simulink model "ofur"  (R2018b)
settings: Solver=VariableStepAuto  StartTime=0.0  StopTime=0.01  RelTol=1e-3
libraries: xbsIndex_r4 x105, commanapbnd3 x4
(part 1 of 2)
settings Model: Creator=IRZ  LastModifiedBy=IRZ

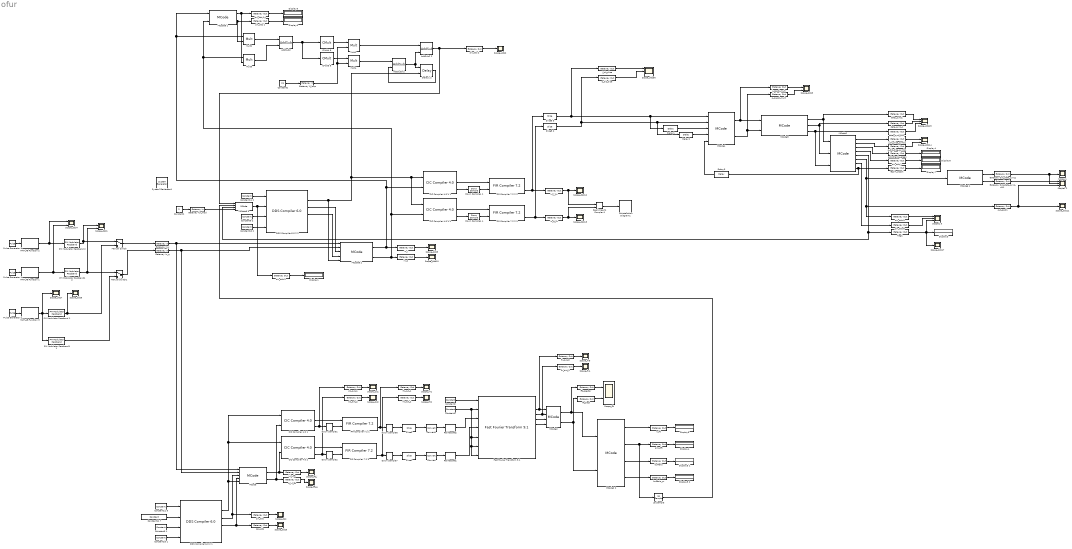
== system ofur ==
  " System Generator1" : xbsIndex_r4/ System Generator  Tag=genX  xilinxfamily=artix7  part=xc7a200t  speed=-3  package=fbg484  synthesis_tool=Vivado  clock_wrapper=Clock Enables  directory=C:/Users/IRZ/AppData/Roaming/Xilinx/Vivado/ofur_24  proj_type=Vivado  Synth_file=Vivado Synthesis Defaults  Impl_file=Vivado Implementation Defaults  testbench=off  simulink_period=1/30.72e6  sysclk_period=32.55  dcm_input_clock_period=10  incr_netlist=off  trim_vbits=Everywhere in SubSystem  dbl_ovrd=According to Block Masks  core_generation=According to Block Masks  run_coregen=off  deprecated_control=off  eval_field=0  block_type=sysgen
  AddSub2 : xbsIndex_r4/AddSub  mode=Subtraction  use_carryin=off  use_carryout=off  en=off  latency=1  precision=Full  arith_type=Unsigned  n_bits=16  bin_pt=14  quantization=Truncate  overflow=Wrap  use_behavioral_HDL=off  hw_selection=Fabric  pipelined=off  dbl_ovrd=off  block_type=addsub
  AddSub2 2 : xbsIndex_r4/AddSub  mode=Addition  use_carryin=off  use_carryout=off  en=off  latency=1  precision=User Defined  arith_type="Signed  (2's comp)"  n_bits=32  bin_pt=32  quantization=Truncate  overflow=Wrap  use_behavioral_HDL=off  hw_selection=Fabric  pipelined=off  dbl_ovrd=off  block_type=addsub
  AddSub3 2 : xbsIndex_r4/AddSub  mode=Addition  use_carryin=off  use_carryout=off  en=off  latency=0  precision=User Defined  arith_type="Signed  (2's comp)"  n_bits=48  bin_pt=48  quantization=Truncate  overflow=Wrap  use_behavioral_HDL=off  hw_selection=Fabric  pipelined=off  dbl_ovrd=off  block_type=addsub
  "CIC Compiler 4.0 1 " : xbsIndex_r4/CIC Compiler 4.0   filter_type=Decimation  number_of_stages=5  differential_delay=1  number_of_channels=1  sample_rate_changes=Fixed  fixed_or_initial_rate=4  minimum_rate=4  maximum_rate=4  ratespecification=Sample_Period  sampleperiod=1  hardwareoversamplingrate=1  quantization=Truncation  output_data_width=24  use_xtreme_dsp_slice=on  use_streaming_interface=on  has_aclken=off  has_aresetn=off  has_dout_tready=off  trim_axipin_name=on  gui_behaviour=Sysgen_GUI  input_data_width=18  ip_name=CIC Compiler  ip_version=4.0  dsptool_ready=true  wrapper_available=true  port_translation_map={ 'aclken' => 'en', 'aresetn' => 'rst' }  ipcore_xco_need_fpga_part=true  ipcore_verbose=false  block_type=cic_compiler_v4_0
  "CIC Compiler 4.0 2 " : xbsIndex_r4/CIC Compiler 4.0   filter_type=Decimation  number_of_stages=5  differential_delay=1  number_of_channels=1  sample_rate_changes=Fixed  fixed_or_initial_rate=4  minimum_rate=4  maximum_rate=4  ratespecification=Sample_Period  sampleperiod=1  hardwareoversamplingrate=1  quantization=Truncation  output_data_width=24  use_xtreme_dsp_slice=on  use_streaming_interface=on  has_aclken=off  has_aresetn=off  has_dout_tready=off  trim_axipin_name=on  gui_behaviour=Sysgen_GUI  input_data_width=18  ip_name=CIC Compiler  ip_version=4.0  dsptool_ready=true  wrapper_available=true  port_translation_map={ 'aclken' => 'en', 'aresetn' => 'rst' }  ipcore_xco_need_fpga_part=true  ipcore_verbose=false  block_type=cic_compiler_v4_0
  CIC Compiler 4.0 4 1 : xbsIndex_r4/CIC Compiler 4.0   filter_type=Decimation  number_of_stages=5  differential_delay=1  number_of_channels=1  sample_rate_changes=Fixed  fixed_or_initial_rate=32  minimum_rate=32  maximum_rate=32  ratespecification=Sample_Period  sampleperiod=1  hardwareoversamplingrate=1  quantization=Truncation  output_data_width=16  use_xtreme_dsp_slice=on  use_streaming_interface=on  has_aclken=off  has_aresetn=off  has_dout_tready=off  trim_axipin_name=on  gui_behaviour=Sysgen_GUI  input_data_width=18  ip_name=CIC Compiler  ip_version=4.0  dsptool_ready=true  wrapper_available=true  port_translation_map={ 'aclken' => 'en', 'aresetn' => 'rst' }  ipcore_xco_need_fpga_part=true  ipcore_verbose=false  block_type=cic_compiler_v4_0
  CIC Compiler 4.0 4 4 : xbsIndex_r4/CIC Compiler 4.0   filter_type=Decimation  number_of_stages=5  differential_delay=1  number_of_channels=1  sample_rate_changes=Fixed  fixed_or_initial_rate=32  minimum_rate=32  maximum_rate=32  ratespecification=Sample_Period  sampleperiod=1  hardwareoversamplingrate=1  quantization=Truncation  output_data_width=16  use_xtreme_dsp_slice=on  use_streaming_interface=on  has_aclken=off  has_aresetn=off  has_dout_tready=off  trim_axipin_name=on  gui_behaviour=Sysgen_GUI  input_data_width=18  ip_name=CIC Compiler  ip_version=4.0  dsptool_ready=true  wrapper_available=true  port_translation_map={ 'aclken' => 'en', 'aresetn' => 'rst' }  ipcore_xco_need_fpga_part=true  ipcore_verbose=false  block_type=cic_compiler_v4_0
  CMult3 5 : xbsIndex_r4/CMult  const=0.00000000010458116751  gui_display_data_type=Fixed-point  const_n_bits=48  const_bin_pt=48  float_type=Single  exp_bits=8  fraction_bits=24  en=off  latency=1  precision=User Defined  arith_type="Signed  (2's comp)"  n_bits=48  bin_pt=48  quantization=Truncate  overflow=Wrap  use_behavioral_HDL=off  mem_type=Distributed RAM  pipeline=off  dbl_ovrd=off  block_type=cmult
  CMult4 5 : xbsIndex_r4/CMult  const=0.0000102265908761675  gui_display_data_type=Fixed-point  const_n_bits=48  const_bin_pt=48  float_type=Single  exp_bits=8  fraction_bits=24  en=off  latency=1  precision=User Defined  arith_type="Signed  (2's comp)"  n_bits=48  bin_pt=48  quantization=Truncate  overflow=Wrap  use_behavioral_HDL=off  mem_type=Distributed RAM  pipeline=off  dbl_ovrd=off  block_type=cmult
  Constant1 : Constant  Value=2
  "Constant1 " : xbsIndex_r4/Constant  const=1.0  gui_display_data_type=Boolean  arith_type=Boolean  n_bits=1  bin_pt=0  preci_type=Single  exp_width=8  frac_width=24  explicit_period=off  period=1/120000  equ=P=C  opselect=C  inp2=PCIN>>17  opr=+  inp1=P  carry=CIN  dbl_ovrd=off  block_type=constant
  Constant10 1 : xbsIndex_r4/Constant  const=1.0  gui_display_data_type=Boolean  arith_type=Boolean  n_bits=16  bin_pt=14  preci_type=Single  exp_width=8  frac_width=24  explicit_period=on  period=1/30.72e6  equ=P=C  opselect=C  inp2=PCIN>>17  opr=+  inp1=P  carry=CIN  dbl_ovrd=off  block_type=constant
  Constant10 2 : xbsIndex_r4/Constant  const=1.0  gui_display_data_type=Boolean  arith_type=Boolean  n_bits=16  bin_pt=14  preci_type=Single  exp_width=8  frac_width=24  explicit_period=on  period=1/30.72e6  equ=P=C  opselect=C  inp2=PCIN>>17  opr=+  inp1=P  carry=CIN  dbl_ovrd=off  block_type=constant
  Constant11 2 : xbsIndex_r4/Constant  const=1.0  gui_display_data_type=Boolean  arith_type=Boolean  n_bits=16  bin_pt=14  preci_type=Single  exp_width=8  frac_width=24  explicit_period=on  period=1/30.72e6  equ=P=C  opselect=C  inp2=PCIN>>17  opr=+  inp1=P  carry=CIN  dbl_ovrd=off  block_type=constant
  Constant11 5 : xbsIndex_r4/Constant  const=1.0  gui_display_data_type=Boolean  arith_type=Boolean  n_bits=16  bin_pt=14  preci_type=Single  exp_width=8  frac_width=24  explicit_period=on  period=1/30.72e6  equ=P=C  opselect=C  inp2=PCIN>>17  opr=+  inp1=P  carry=CIN  dbl_ovrd=off  block_type=constant
  Constant11 7 : xbsIndex_r4/Constant  const=0.03255208333333  gui_display_data_type=Fixed-point  arith_type=Unsigned  n_bits=32  bin_pt=32  preci_type=Single  exp_width=8  frac_width=24  explicit_period=on  period=1/30.72e6  equ=P=C  opselect=C  inp2=PCIN>>17  opr=+  inp1=P  carry=CIN  dbl_ovrd=off  block_type=constant
  Constant2 : Constant  Value=24
  "Constant2 " : xbsIndex_r4/Constant  const=1.0  gui_display_data_type=Fixed-point  arith_type=Unsigned  n_bits=1  bin_pt=0  preci_type=Single  exp_width=8  frac_width=24  explicit_period=off  period=1/120000  equ=P=C  opselect=C  inp2=PCIN>>17  opr=+  inp1=P  carry=CIN  dbl_ovrd=off  block_type=constant
  Constant9 1 : xbsIndex_r4/Constant  const=1.0  gui_display_data_type=Boolean  arith_type=Boolean  n_bits=16  bin_pt=14  preci_type=Single  exp_width=8  frac_width=24  explicit_period=on  period=1/30.72e6  equ=P=C  opselect=C  inp2=PCIN>>17  opr=+  inp1=P  carry=CIN  dbl_ovrd=off  block_type=constant
  Constant9 2 : xbsIndex_r4/Constant  const=1.0  gui_display_data_type=Boolean  arith_type=Boolean  n_bits=16  bin_pt=14  preci_type=Single  exp_width=8  frac_width=24  explicit_period=on  period=1/30.72e6  equ=P=C  opselect=C  inp2=PCIN>>17  opr=+  inp1=P  carry=CIN  dbl_ovrd=off  block_type=constant
  Constellation Diagram1 : ConstellationDiagram
  "Convert " : xbsIndex_r4/Convert  gui_display_data_type=Fixed-point  arith_type="Signed  (2's comp)"  n_bits=21  bin_pt=0  float_type=Single  exp_bits=8  fraction_bits=24  quantization=Truncate  overflow=Wrap  en=off  latency=0  pipeline=off  dbl_ovrd=off  block_type=convert
  "Convert1 " : xbsIndex_r4/Convert  gui_display_data_type=Fixed-point  arith_type="Signed  (2's comp)"  n_bits=21  bin_pt=0  float_type=Single  exp_bits=8  fraction_bits=24  quantization=Truncate  overflow=Wrap  en=off  latency=0  pipeline=off  dbl_ovrd=off  block_type=convert
  DDS Compiler 6.0 2 1 : xbsIndex_r4/DDS Compiler 6.0   partspresent=Phase_Generator_and_SIN_COS_LUT  dds_clock_rate=30.72  channels=1  mode_of_operation=Standard  modulus=9  parameter_entry=Hardware_Parameters  spurious_free_dynamic_range=45  frequency_resolution=0.4  noise_shaping=None  phase_width=32  output_width=12  output_selection=Sine_and_Cosine  negative_sine=on  negative_cosine=on  amplitude_mode=Full_Range  memory_type=Auto  optimization_goal=Auto  dsp48_use=Minimal  resync=off  latency_configuration=Auto  latency=1  has_phase_out=on  has_aclken=off  has_aresetn=off  explicit_period=on  period=1/30.72e6  data_has_tlast=Not_Required  has_tready=on  s_phase_has_tuser=Not_Required  m_data_has_tuser=Not_Required  m_phase_has_tuser=Not_Required  s_phase_tuser_width=1  output_form=Twos_Complement  s_config_sync_mode=On_Vector  phase_increment=Streaming  output_frequency1=0  output_frequency2=0  output_frequency3=0  output_frequency4=0  output_frequency5=0  output_frequency6=0  output_frequency7=0  output_frequency8=0  output_frequency9=0  output_frequency10=0  output_frequency11=0  output_frequency12=0  output_frequency13=0  output_frequency14=0  output_frequency15=0  output_frequency16=0  pinc1='0'  pinc2='0'  pinc3='0'  pinc4='0'  pinc5='0'  pinc6='0'  pinc7='0'  pinc8='0'  pinc9='0'  pinc10='0'  pinc11='0'  pinc12='0'  pinc13='0'  pinc14='0'  pinc15='0'  pinc16='0'  phase_offset=Fixed  phase_offset_angles1=0  phase_offset_angles2=0  phase_offset_angles3=0  phase_offset_angles4=0  phase_offset_angles5=0  phase_offset_angles6=0  phase_offset_angles7=0  phase_offset_angles8=0  phase_offset_angles9=0  phase_offset_angles10=0  phase_offset_angles11=0  phase_offset_angles12=0  phase_offset_angles13=0  phase_offset_angles14=0  phase_offset_angles15=0  phase_offset_angles16=0  poff1='0'  poff2='0'  poff3='0'  poff4='0'  poff5='0'  poff6='0'  poff7='0'  poff8='0'  poff9='0'  poff10='0'  poff11='0'  poff12='0'  poff13='0'  poff14='0'  poff15='0'  poff16='0'  trim_axipin_name=on  simulation_type=hybrid_sim  simulation_model=sysgen:xddsv6_0_cmodel  data_path_portlist={ 's_axis_config_tdata_poff', 's_axis_config_tdata_chan0_poff', 's_axis_config_tdata_pinc', 's_axis_config_tdata_chan0_pinc', 's_axis_phase_tdata_resync', 's_axis_phase_tdata_chan0_resync', 's_axis_phase_tdata_poff', 's_axis_phase_tdata_chan0_poff', 's_axis_phase_tdata_pinc', 's_axis_phase_tdata_chan0_pinc', 's_axis_phase_tdata_phase_in', 'm_axis_data_tdata_sine', 'm_axis_data_tdata_chan0_sine', 'm_axis_data_tdata_cosine', 'm_axis_data_tdata_chan0_cosine', 'm_axis_phase_tdata_phase_out', 'm_axis_phase_tdata_chan0_phase_out'}  por_mode=false  gui_behaviour=Sysgen  ip_name=DDS Compiler  ip_version=6.0  dsptool_ready=true  wrapper_available=true  port_translation_map={ 'aclken' => 'en', 'aresetn' => 'rst' }  ipcore_usecache=true  ipcore_useipmodelcache=true  ipcore_xco_need_fpga_part=true  ipcore_verbose=false  block_type=dds_compiler_v6_0
  DDS Compiler 6.0 2 2 : xbsIndex_r4/DDS Compiler 6.0   partspresent=Phase_Generator_and_SIN_COS_LUT  dds_clock_rate=30.72  channels=1  mode_of_operation=Standard  modulus=9  parameter_entry=Hardware_Parameters  spurious_free_dynamic_range=45  frequency_resolution=0.4  noise_shaping=None  phase_width=32  output_width=12  output_selection=Sine_and_Cosine  negative_sine=on  negative_cosine=on  amplitude_mode=Full_Range  memory_type=Auto  optimization_goal=Auto  dsp48_use=Minimal  resync=off  latency_configuration=Auto  latency=1  has_phase_out=on  has_aclken=off  has_aresetn=off  explicit_period=on  period=1/30.72e6  data_has_tlast=Not_Required  has_tready=on  s_phase_has_tuser=Not_Required  m_data_has_tuser=Not_Required  m_phase_has_tuser=Not_Required  s_phase_tuser_width=1  output_form=Twos_Complement  s_config_sync_mode=On_Vector  phase_increment=Streaming  output_frequency1=0  output_frequency2=0  output_frequency3=0  output_frequency4=0  output_frequency5=0  output_frequency6=0  output_frequency7=0  output_frequency8=0  output_frequency9=0  output_frequency10=0  output_frequency11=0  output_frequency12=0  output_frequency13=0  output_frequency14=0  output_frequency15=0  output_frequency16=0  pinc1='0'  pinc2='0'  pinc3='0'  pinc4='0'  pinc5='0'  pinc6='0'  pinc7='0'  pinc8='0'  pinc9='0'  pinc10='0'  pinc11='0'  pinc12='0'  pinc13='0'  pinc14='0'  pinc15='0'  pinc16='0'  phase_offset=Fixed  phase_offset_angles1=0  phase_offset_angles2=0  phase_offset_angles3=0  phase_offset_angles4=0  phase_offset_angles5=0  phase_offset_angles6=0  phase_offset_angles7=0  phase_offset_angles8=0  phase_offset_angles9=0  phase_offset_angles10=0  phase_offset_angles11=0  phase_offset_angles12=0  phase_offset_angles13=0  phase_offset_angles14=0  phase_offset_angles15=0  phase_offset_angles16=0  poff1='0'  poff2='0'  poff3='0'  poff4='0'  poff5='0'  poff6='0'  poff7='0'  poff8='0'  poff9='0'  poff10='0'  poff11='0'  poff12='0'  poff13='0'  poff14='0'  poff15='0'  poff16='0'  trim_axipin_name=on  simulation_type=hybrid_sim  simulation_model=sysgen:xddsv6_0_cmodel  data_path_portlist={ 's_axis_config_tdata_poff', 's_axis_config_tdata_chan0_poff', 's_axis_config_tdata_pinc', 's_axis_config_tdata_chan0_pinc', 's_axis_phase_tdata_resync', 's_axis_phase_tdata_chan0_resync', 's_axis_phase_tdata_poff', 's_axis_phase_tdata_chan0_poff', 's_axis_phase_tdata_pinc', 's_axis_phase_tdata_chan0_pinc', 's_axis_phase_tdata_phase_in', 'm_axis_data_tdata_sine', 'm_axis_data_tdata_chan0_sine', 'm_axis_data_tdata_cosine', 'm_axis_data_tdata_chan0_cosine', 'm_axis_phase_tdata_phase_out', 'm_axis_phase_tdata_chan0_phase_out'}  por_mode=false  gui_behaviour=Sysgen  ip_name=DDS Compiler  ip_version=6.0  dsptool_ready=true  wrapper_available=true  port_translation_map={ 'aclken' => 'en', 'aresetn' => 'rst' }  ipcore_usecache=true  ipcore_useipmodelcache=true  ipcore_xco_need_fpga_part=true  ipcore_verbose=false  block_type=dds_compiler_v6_0
  Delay1 : xbsIndex_r4/Delay  rst=off  infoeditControl=Selection of Reset will increase slice count due to use of real FFs and instead of SRLs  en=off  latency=60  reg_retiming=off  dbl_ovrd=off  block_type=delay
  Delay1 2 : xbsIndex_r4/Delay  rst=off  infoeditControl=Selection of Reset will increase slice count due to use of real FFs and instead of SRLs  en=on  latency=1  reg_retiming=off  dbl_ovrd=off  block_type=delay
  Delay2 : xbsIndex_r4/Delay  rst=off  infoeditControl=Selection of Reset will increase slice count due to use of real FFs and instead of SRLs  en=off  latency=60  reg_retiming=off  dbl_ovrd=off  block_type=delay
  Delay3 : xbsIndex_r4/Delay  rst=off  infoeditControl=Selection of Reset will increase slice count due to use of real FFs and instead of SRLs  en=off  latency=1  reg_retiming=off  dbl_ovrd=off  block_type=delay
  Display{1,3..8} (7 alike) : Display
  "Display4 " : Display
  "Display5 " : Display
  Display5 1 : Display
  Display5 2 : Display
  "Down Sample1 " : xbsIndex_r4/Down Sample  sample_ratio=4  sample_phase="Last Value of Frame  (most efficient)"  en=off  rst=off  latency=1  dbl_ovrd=off  block_type=dsamp
  "Down Sample2 " : xbsIndex_r4/Down Sample  sample_ratio=4  sample_phase="Last Value of Frame  (most efficient)"  en=off  rst=off  latency=1  dbl_ovrd=off  block_type=dsamp
  Down Sample4 1 : xbsIndex_r4/Down Sample  sample_ratio=32  sample_phase="Last Value of Frame  (most efficient)"  en=off  rst=off  latency=1  dbl_ovrd=off  block_type=dsamp
  Down Sample4 4 : xbsIndex_r4/Down Sample  sample_ratio=32  sample_phase="Last Value of Frame  (most efficient)"  en=off  rst=off  latency=1  dbl_ovrd=off  block_type=dsamp
  "Down Sample6 " : xbsIndex_r4/Down Sample  sample_ratio=4  sample_phase="Last Value of Frame  (most efficient)"  en=off  rst=off  latency=1  dbl_ovrd=off  block_type=dsamp
  "Down Sample7 " : xbsIndex_r4/Down Sample  sample_ratio=4  sample_phase="Last Value of Frame  (most efficient)"  en=off  rst=off  latency=1  dbl_ovrd=off  block_type=dsamp
  "FIR Compiler 7.2 1 " : xbsIndex_r4/FIR Compiler 7.2   coefficientvector=[5961,-4341,-5200,5397,4251,-6331,-3141,7100,1875,-7671,-458,8028,-1084,-8145,2709,7981,-4390,-7515,6071,6714,-7711,-5578,9238,4098,-10576,-2278,11650,136,-12393,2277,12717,-4911,-12561,7674,11849,-10487,-10548,13229,8632,-15771,-6099,17971,2967,-19698,699,20806,-4819,-21177,9255,20681,-13870,-19237,18484,16792,-22893,-13332,26871,8872,-30202,-3496,32654,-2687,-34033,9480,34134,-16674,-32809,24007,29954,-31182,-25527,37863,19534,-43720,-12068,48399,3266,-51603,6615,53018,-17279,-52399,28360,49556,-39446,-44391,50062,36877,-59727,-27101,67922,15214,-74196,-1526,78087,-13579,-79202,29613,77220,-46023,-71936,62164,63244,-77368,-51198,90890,35929,-102064,-17776,110212,-2802,-114730,25190,115084,-48675,-110890,72410,101880,-95502,-88017,116918,69351,-135693,-46197,150834,19045,-161429,11387,166618,-44226,-165712,78400,158145,-112759,-143659,145915,122105,-176513,-93664,203106,58734,-224327,-18056,238810,-27410,-245362,76380,242864,-127466,-230591,178883,207912,-228803,-174609,275166,130682,-315950,-76603,348997,13114,-372286,58521,383660,-136955,-381405,220191,363720,-306141,-329247,392180,276603,-475673,-204895,553510,113191,-622681,-1152,679399,-132151,-720279,287147,740942,-465392,-737162,668670,702872,-901701,-631137,1172158,510308,-1497574,-323934,1911126,37391,-2496341,416174,3480027,-1210770,-5782518,2698242,16777215,16777215,2698242,-5782518,-1210770,3480027,416174,-2496341,37391,1911126,-323934,-1497574,510308,1172158,-631137,-901701,702872,668670,-737162,-465392,740942,287147,-720279,-132151,679399,-1152,-622681,113191,553510,-204895,-475673,276603,392180,-329247,-306141,363720,220191,-381405,-136955,383660,58521,-372286,13114,348997,-76603,-315950,130682,275166,-174609,-228803,207912,178883,-230591,-127466,242864,76380,-245362,-27410,238810,-18056,-224327,58734,203106,-93664,-176513,122105,145915,-143659,-112759,158145,78400,-165712,-44226,166618,11387,-161429,19045,150834,-46197,-135693,69351,116918,-88017,-95502,101880,72410,-110890,-48675,115084,25190,-114730,-2802,110212,-17776,-102064,35929,90890,-51198,-77368,63244,62164,-71936,-46023,77220,29613,-79202,-13579,78087,-1526,-74196,15214,67922,-27101,-59727,36877,50062,-44391,-39446,49556,28360,-52399,-17279,53018,6615,-51603,3266,48399,-12068,-43720,19534,37863,-25527,-31182,29954,24007,-32809,-16674,34134,9480,-34033,-2687,32654,-3496,-30202,8872,26871,-13332,-22893,16792,18484,-19237,-13870,20681,9255,-21177,-4819,20806,699,-19698,2967,17971,-6099,-15771,8632,13229,-10548,-10487,11849,7674,-12561,-4911,12717,2277,-12393,136,11650,-2278,-10576,4098,9238,-5578,-7711,6714,6071,-7515,-4390,7981,2709,-8145,-1084,8028,-458,-7671,1875,7100,-3141,-6331,4251,5397,-5200,-4341,5961]  coefficient_sets=1  coefficient_reload=off  filter_type=Single_Rate  rate_change_type=Integer  interpolation_rate=1  decimation_rate=1  zero_pack_factor=1  channel_sequence=Basic  number_channels=1  pattern_list='P4-0,P4-1,P4-2,P4-3,P4-4'  number_paths=1  ratespecification=Input_Sample_Period  sampleperiod=4  hardwareoversamplingrate=1  coefficient_sign=Signed  quantization=Integer_Coefficients  coefficient_width=25  bestprecision=off  coefficient_fractional_bits=0  coefficient_structure=Inferred  output_rounding_mode=Truncate_LSBs  output_width=24  filter_architecture=Systolic_Multiply_Accumulate  optimization_goal=Area  optimization_list='None'  data_buffer_type=Automatic  coefficient_buffer_type=Automatic  input_buffer_type=Automatic  output_buffer_type=Automatic  preference_for_other_storage=Automatic  multi_column_support=Automatic  columnconfig='51'  inter_column_pipe_length=4  data_has_tlast=Not_Required  m_data_has_tready=off  s_data_has_fifo=off  s_data_has_tuser=Not_Required  m_data_has_tuser=Not_Required  s_config_sync_mode=On_Vector  s_config_method=Single  num_reload_slots=1  has_aclken=off  has_aresetn=off  infoeditControl=ARESETn must be asserted for a minimum of 2 cycles  reset_data_vector=on  trim_axipin_name=on  simulation_type=hybrid_sim  simulation_model=sysgen:xfirv7_2_cmodel  data_path_portlist={ 's_axis_data_tdata', 'm_axis_data_tdata' }  passband_min=0.0  passband_max=0.5  stopband_min=0.5  stopband_max=1.0  filter_selection=1  gui_behaviour='Sysgen_GUI'  data_sign=Signed  data_width=16  data_fractional_bits=0  data_tuser_width=1  wrapper_available=true  ip_wrap_arbitrary_binary_point=true  ip_name=FIR Compiler  ip_version=7.2  dsptool_ready=true  ipcore_usecache=true  ipcore_useipmodelcache=true  port_translation_map={ 'aclken' => 'en', 'aresetn' => 'rst' }  run_core_at_system_period=true  ipcore_xco_need_fpga_part=true  block_type=fir_compiler_v7_2
      settings: infoedit=Maximum Possible : Maximizes oversampling rate. Abstracted input handshake (no s_data_tvalid) and automatic rate propagation.<br>Hardware Oversampling Rate : Specifies oversampling rate relative to the input sample period. Abstracted input handshake (no s_data_tvalid) and automatic rate propagation.<br>Input/Output Sample Period : Specifies absolute oversampling rate. No input handshake abstraction (exposes s_data_tvalid) and no rate propagation.
  FIR Compiler 7.2 2 1 : xbsIndex_r4/FIR Compiler 7.2   coefficientvector=[5553,-5324,-4273,6479,2702,-7305,-920,7729,-1006,-7701,3003,7201,-4966,-6223,6772,4761,-8314,-2856,9463,560,-10121,2017,10174,-4751,-9540,7488,8172,-10055,-6076,12244,3285,-13863,90,14710,-3911,-14639,7955,13523,-11964,-11299,15648,7970,-18710,-3641,20835,-1519,-21758,7231,21238,-13176,-19143,18942,15423,-24088,-10141,28160,3476,-30743,4251,31459,-12621,-30047,21090,26330,-29083,-20322,35967,12188,-41120,-2270,43970,-8936,-44066,20767,41089,-32467,-34935,43163,25668,-52014,-13621,58198,-650,-61006,16364,59879,-32580,-54501,48204,44804,-62111,-31063,73124,13805,-80206,6116,82482,-27581,-79334,49244,70445,-69637,-55886,87221,36094,-100558,-11978,108295,-15238,-109384,43981,103126,-72441,-89280,98635,68072,-120580,-40278,136365,7130,-144406,29567,143406,-67681,-132608,104757,111814,-138224,-81521,165478,42865,-184127,2310,192056,-51669,-187798,102250,170439,-150824,-139900,193936,96894,-228227,-43078,250533,-19090,-258224,86280,249201,-154701,-222419,219925,177699,-277402,-116076,322477,39610,-350898,48399,358869,-143713,-343561,240967,302909,-334404,-236394,417533,144637,-483910,-29968,526925,-104076,-540617,252289,519407,-408479,-459016,564715,355472,-712754,-206430,842864,9618,-945294,236166,1008549,-533823,-1020728,888019,965947,-1312331,-824719,1835158,561006,-2534935,-109960,3632892,-689814,-6037165,2102535,16777215,16777215,2102535,-6037165,-689814,3632892,-109960,-2534935,561006,1835158,-824719,-1312331,965947,888019,-1020728,-533823,1008549,236166,-945294,9618,842864,-206430,-712754,355472,564715,-459016,-408479,519407,252289,-540617,-104076,526925,-29968,-483910,144637,417533,-236394,-334404,302909,240967,-343561,-143713,358869,48399,-350898,39610,322477,-116076,-277402,177699,219925,-222419,-154701,249201,86280,-258224,-19090,250533,-43078,-228227,96894,193936,-139900,-150824,170439,102250,-187798,-51669,192056,2310,-184127,42865,165478,-81521,-138224,111814,104757,-132608,-67681,143406,29567,-144406,7130,136365,-40278,-120580,68072,98635,-89280,-72441,103126,43981,-109384,-15238,108295,-11978,-100558,36094,87221,-55886,-69637,70445,49244,-79334,-27581,82482,6116,-80206,13805,73124,-31063,-62111,44804,48204,-54501,-32580,59879,16364,-61006,-650,58198,-13621,-52014,25668,43163,-34935,-32467,41089,20767,-44066,-8936,43970,-2270,-41120,12188,35967,-20322,-29083,26330,21090,-30047,-12621,31459,4251,-30743,3476,28160,-10141,-24088,15423,18942,-19143,-13176,21238,7231,-21758,-1519,20835,-3641,-18710,7970,15648,-11299,-11964,13523,7955,-14639,-3911,14710,90,-13863,3285,12244,-6076,-10055,8172,7488,-9540,-4751,10174,2017,-10121,560,9463,-2856,-8314,4761,6772,-6223,-4966,7201,3003,-7701,-1006,7729,-920,-7305,2702,6479,-4273,-5324,5553]  coefficient_sets=1  coefficient_reload=off  filter_type=Single_Rate  rate_change_type=Integer  interpolation_rate=1  decimation_rate=1  zero_pack_factor=1  channel_sequence=Basic  number_channels=1  pattern_list='P4-0,P4-1,P4-2,P4-3,P4-4'  number_paths=1  ratespecification=Input_Sample_Period  sampleperiod=32  hardwareoversamplingrate=1  coefficient_sign=Signed  quantization=Integer_Coefficients  coefficient_width=25  bestprecision=off  coefficient_fractional_bits=0  coefficient_structure=Inferred  output_rounding_mode=Truncate_LSBs  output_width=16  filter_architecture=Systolic_Multiply_Accumulate  optimization_goal=Area  optimization_list='None'  data_buffer_type=Automatic  coefficient_buffer_type=Automatic  input_buffer_type=Automatic  output_buffer_type=Automatic  preference_for_other_storage=Automatic  multi_column_support=Automatic  columnconfig='7'  inter_column_pipe_length=4  data_has_tlast=Not_Required  m_data_has_tready=off  s_data_has_fifo=off  s_data_has_tuser=Not_Required  m_data_has_tuser=Not_Required  s_config_sync_mode=On_Vector  s_config_method=Single  num_reload_slots=1  has_aclken=off  has_aresetn=off  infoeditControl=ARESETn must be asserted for a minimum of 2 cycles  reset_data_vector=on  trim_axipin_name=on  simulation_type=hybrid_sim  simulation_model=sysgen:xfirv7_2_cmodel  data_path_portlist={ 's_axis_data_tdata', 'm_axis_data_tdata' }  passband_min=0.0  passband_max=0.5  stopband_min=0.5  stopband_max=1.0  filter_selection=1  gui_behaviour='Sysgen_GUI'  data_sign=Signed  data_width=16  data_fractional_bits=0  data_tuser_width=1  wrapper_available=true  ip_wrap_arbitrary_binary_point=true  ip_name=FIR Compiler  ip_version=7.2  dsptool_ready=true  ipcore_usecache=true  ipcore_useipmodelcache=true  port_translation_map={ 'aclken' => 'en', 'aresetn' => 'rst' }  run_core_at_system_period=true  ipcore_xco_need_fpga_part=true  block_type=fir_compiler_v7_2
      settings: infoedit=Maximum Possible : Maximizes oversampling rate. Abstracted input handshake (no s_data_tvalid) and automatic rate propagation.<br>Hardware Oversampling Rate : Specifies oversampling rate relative to the input sample period. Abstracted input handshake (no s_data_tvalid) and automatic rate propagation.<br>Input/Output Sample Period : Specifies absolute oversampling rate. No input handshake abstraction (exposes s_data_tvalid) and no rate propagation.
  FIR Compiler 7.2 2 4 : xbsIndex_r4/FIR Compiler 7.2   coefficientvector=[5553,-5324,-4273,6479,2702,-7305,-920,7729,-1006,-7701,3003,7201,-4966,-6223,6772,4761,-8314,-2856,9463,560,-10121,2017,10174,-4751,-9540,7488,8172,-10055,-6076,12244,3285,-13863,90,14710,-3911,-14639,7955,13523,-11964,-11299,15648,7970,-18710,-3641,20835,-1519,-21758,7231,21238,-13176,-19143,18942,15423,-24088,-10141,28160,3476,-30743,4251,31459,-12621,-30047,21090,26330,-29083,-20322,35967,12188,-41120,-2270,43970,-8936,-44066,20767,41089,-32467,-34935,43163,25668,-52014,-13621,58198,-650,-61006,16364,59879,-32580,-54501,48204,44804,-62111,-31063,73124,13805,-80206,6116,82482,-27581,-79334,49244,70445,-69637,-55886,87221,36094,-100558,-11978,108295,-15238,-109384,43981,103126,-72441,-89280,98635,68072,-120580,-40278,136365,7130,-144406,29567,143406,-67681,-132608,104757,111814,-138224,-81521,165478,42865,-184127,2310,192056,-51669,-187798,102250,170439,-150824,-139900,193936,96894,-228227,-43078,250533,-19090,-258224,86280,249201,-154701,-222419,219925,177699,-277402,-116076,322477,39610,-350898,48399,358869,-143713,-343561,240967,302909,-334404,-236394,417533,144637,-483910,-29968,526925,-104076,-540617,252289,519407,-408479,-459016,564715,355472,-712754,-206430,842864,9618,-945294,236166,1008549,-533823,-1020728,888019,965947,-1312331,-824719,1835158,561006,-2534935,-109960,3632892,-689814,-6037165,2102535,16777215,16777215,2102535,-6037165,-689814,3632892,-109960,-2534935,561006,1835158,-824719,-1312331,965947,888019,-1020728,-533823,1008549,236166,-945294,9618,842864,-206430,-712754,355472,564715,-459016,-408479,519407,252289,-540617,-104076,526925,-29968,-483910,144637,417533,-236394,-334404,302909,240967,-343561,-143713,358869,48399,-350898,39610,322477,-116076,-277402,177699,219925,-222419,-154701,249201,86280,-258224,-19090,250533,-43078,-228227,96894,193936,-139900,-150824,170439,102250,-187798,-51669,192056,2310,-184127,42865,165478,-81521,-138224,111814,104757,-132608,-67681,143406,29567,-144406,7130,136365,-40278,-120580,68072,98635,-89280,-72441,103126,43981,-109384,-15238,108295,-11978,-100558,36094,87221,-55886,-69637,70445,49244,-79334,-27581,82482,6116,-80206,13805,73124,-31063,-62111,44804,48204,-54501,-32580,59879,16364,-61006,-650,58198,-13621,-52014,25668,43163,-34935,-32467,41089,20767,-44066,-8936,43970,-2270,-41120,12188,35967,-20322,-29083,26330,21090,-30047,-12621,31459,4251,-30743,3476,28160,-10141,-24088,15423,18942,-19143,-13176,21238,7231,-21758,-1519,20835,-3641,-18710,7970,15648,-11299,-11964,13523,7955,-14639,-3911,14710,90,-13863,3285,12244,-6076,-10055,8172,7488,-9540,-4751,10174,2017,-10121,560,9463,-2856,-8314,4761,6772,-6223,-4966,7201,3003,-7701,-1006,7729,-920,-7305,2702,6479,-4273,-5324,5553]  coefficient_sets=1  coefficient_reload=off  filter_type=Single_Rate  rate_change_type=Integer  interpolation_rate=1  decimation_rate=1  zero_pack_factor=1  channel_sequence=Basic  number_channels=1  pattern_list='P4-0,P4-1,P4-2,P4-3,P4-4'  number_paths=1  ratespecification=Input_Sample_Period  sampleperiod=32  hardwareoversamplingrate=1  coefficient_sign=Signed  quantization=Integer_Coefficients  coefficient_width=25  bestprecision=off  coefficient_fractional_bits=0  coefficient_structure=Inferred  output_rounding_mode=Truncate_LSBs  output_width=16  filter_architecture=Systolic_Multiply_Accumulate  optimization_goal=Area  optimization_list='None'  data_buffer_type=Automatic  coefficient_buffer_type=Automatic  input_buffer_type=Automatic  output_buffer_type=Automatic  preference_for_other_storage=Automatic  multi_column_support=Automatic  columnconfig='7'  inter_column_pipe_length=4  data_has_tlast=Not_Required  m_data_has_tready=off  s_data_has_fifo=off  s_data_has_tuser=Not_Required  m_data_has_tuser=Not_Required  s_config_sync_mode=On_Vector  s_config_method=Single  num_reload_slots=1  has_aclken=off  has_aresetn=off  infoeditControl=ARESETn must be asserted for a minimum of 2 cycles  reset_data_vector=on  trim_axipin_name=on  simulation_type=hybrid_sim  simulation_model=sysgen:xfirv7_2_cmodel  data_path_portlist={ 's_axis_data_tdata', 'm_axis_data_tdata' }  passband_min=0.0  passband_max=0.5  stopband_min=0.5  stopband_max=1.0  filter_selection=1  gui_behaviour='Sysgen_GUI'  data_sign=Signed  data_width=16  data_fractional_bits=0  data_tuser_width=1  wrapper_available=true  ip_wrap_arbitrary_binary_point=true  ip_name=FIR Compiler  ip_version=7.2  dsptool_ready=true  ipcore_usecache=true  ipcore_useipmodelcache=true  port_translation_map={ 'aclken' => 'en', 'aresetn' => 'rst' }  run_core_at_system_period=true  ipcore_xco_need_fpga_part=true  block_type=fir_compiler_v7_2
      settings: infoedit=Maximum Possible : Maximizes oversampling rate. Abstracted input handshake (no s_data_tvalid) and automatic rate propagation.<br>Hardware Oversampling Rate : Specifies oversampling rate relative to the input sample period. Abstracted input handshake (no s_data_tvalid) and automatic rate propagation.<br>Input/Output Sample Period : Specifies absolute oversampling rate. No input handshake abstraction (exposes s_data_tvalid) and no rate propagation.
  "FIR Compiler 7.2 3 " : xbsIndex_r4/FIR Compiler 7.2   coefficientvector=[5961,-4341,-5200,5397,4251,-6331,-3141,7100,1875,-7671,-458,8028,-1084,-8145,2709,7981,-4390,-7515,6071,6714,-7711,-5578,9238,4098,-10576,-2278,11650,136,-12393,2277,12717,-4911,-12561,7674,11849,-10487,-10548,13229,8632,-15771,-6099,17971,2967,-19698,699,20806,-4819,-21177,9255,20681,-13870,-19237,18484,16792,-22893,-13332,26871,8872,-30202,-3496,32654,-2687,-34033,9480,34134,-16674,-32809,24007,29954,-31182,-25527,37863,19534,-43720,-12068,48399,3266,-51603,6615,53018,-17279,-52399,28360,49556,-39446,-44391,50062,36877,-59727,-27101,67922,15214,-74196,-1526,78087,-13579,-79202,29613,77220,-46023,-71936,62164,63244,-77368,-51198,90890,35929,-102064,-17776,110212,-2802,-114730,25190,115084,-48675,-110890,72410,101880,-95502,-88017,116918,69351,-135693,-46197,150834,19045,-161429,11387,166618,-44226,-165712,78400,158145,-112759,-143659,145915,122105,-176513,-93664,203106,58734,-224327,-18056,238810,-27410,-245362,76380,242864,-127466,-230591,178883,207912,-228803,-174609,275166,130682,-315950,-76603,348997,13114,-372286,58521,383660,-136955,-381405,220191,363720,-306141,-329247,392180,276603,-475673,-204895,553510,113191,-622681,-1152,679399,-132151,-720279,287147,740942,-465392,-737162,668670,702872,-901701,-631137,1172158,510308,-1497574,-323934,1911126,37391,-2496341,416174,3480027,-1210770,-5782518,2698242,16777215,16777215,2698242,-5782518,-1210770,3480027,416174,-2496341,37391,1911126,-323934,-1497574,510308,1172158,-631137,-901701,702872,668670,-737162,-465392,740942,287147,-720279,-132151,679399,-1152,-622681,113191,553510,-204895,-475673,276603,392180,-329247,-306141,363720,220191,-381405,-136955,383660,58521,-372286,13114,348997,-76603,-315950,130682,275166,-174609,-228803,207912,178883,-230591,-127466,242864,76380,-245362,-27410,238810,-18056,-224327,58734,203106,-93664,-176513,122105,145915,-143659,-112759,158145,78400,-165712,-44226,166618,11387,-161429,19045,150834,-46197,-135693,69351,116918,-88017,-95502,101880,72410,-110890,-48675,115084,25190,-114730,-2802,110212,-17776,-102064,35929,90890,-51198,-77368,63244,62164,-71936,-46023,77220,29613,-79202,-13579,78087,-1526,-74196,15214,67922,-27101,-59727,36877,50062,-44391,-39446,49556,28360,-52399,-17279,53018,6615,-51603,3266,48399,-12068,-43720,19534,37863,-25527,-31182,29954,24007,-32809,-16674,34134,9480,-34033,-2687,32654,-3496,-30202,8872,26871,-13332,-22893,16792,18484,-19237,-13870,20681,9255,-21177,-4819,20806,699,-19698,2967,17971,-6099,-15771,8632,13229,-10548,-10487,11849,7674,-12561,-4911,12717,2277,-12393,136,11650,-2278,-10576,4098,9238,-5578,-7711,6714,6071,-7515,-4390,7981,2709,-8145,-1084,8028,-458,-7671,1875,7100,-3141,-6331,4251,5397,-5200,-4341,5961]  coefficient_sets=1  coefficient_reload=off  filter_type=Single_Rate  rate_change_type=Integer  interpolation_rate=1  decimation_rate=1  zero_pack_factor=1  channel_sequence=Basic  number_channels=1  pattern_list='P4-0,P4-1,P4-2,P4-3,P4-4'  number_paths=1  ratespecification=Input_Sample_Period  sampleperiod=4  hardwareoversamplingrate=1  coefficient_sign=Signed  quantization=Integer_Coefficients  coefficient_width=25  bestprecision=off  coefficient_fractional_bits=0  coefficient_structure=Inferred  output_rounding_mode=Truncate_LSBs  output_width=24  filter_architecture=Systolic_Multiply_Accumulate  optimization_goal=Area  optimization_list='None'  data_buffer_type=Automatic  coefficient_buffer_type=Automatic  input_buffer_type=Automatic  output_buffer_type=Automatic  preference_for_other_storage=Automatic  multi_column_support=Automatic  columnconfig='51'  inter_column_pipe_length=4  data_has_tlast=Not_Required  m_data_has_tready=off  s_data_has_fifo=off  s_data_has_tuser=Not_Required  m_data_has_tuser=Not_Required  s_config_sync_mode=On_Vector  s_config_method=Single  num_reload_slots=1  has_aclken=off  has_aresetn=off  infoeditControl=ARESETn must be asserted for a minimum of 2 cycles  reset_data_vector=on  trim_axipin_name=on  simulation_type=hybrid_sim  simulation_model=sysgen:xfirv7_2_cmodel  data_path_portlist={ 's_axis_data_tdata', 'm_axis_data_tdata' }  passband_min=0.0  passband_max=0.5  stopband_min=0.5  stopband_max=1.0  filter_selection=1  gui_behaviour='Sysgen_GUI'  data_sign=Signed  data_width=16  data_fractional_bits=0  data_tuser_width=1  wrapper_available=true  ip_wrap_arbitrary_binary_point=true  ip_name=FIR Compiler  ip_version=7.2  dsptool_ready=true  ipcore_usecache=true  ipcore_useipmodelcache=true  port_translation_map={ 'aclken' => 'en', 'aresetn' => 'rst' }  run_core_at_system_period=true  ipcore_xco_need_fpga_part=true  block_type=fir_compiler_v7_2
      settings: infoedit=Maximum Possible : Maximizes oversampling rate. Abstracted input handshake (no s_data_tvalid) and automatic rate propagation.<br>Hardware Oversampling Rate : Specifies oversampling rate relative to the input sample period. Abstracted input handshake (no s_data_tvalid) and automatic rate propagation.<br>Input/Output Sample Period : Specifies absolute oversampling rate. No input handshake abstraction (exposes s_data_tvalid) and no rate propagation.
  "Fast Fourier Transform 9.1 " : xbsIndex_r4/Fast Fourier Transform 9.1   transform_length=2048  target_clock_frequency=1  target_data_throughput=50  implementation_options=pipelined_streaming_io  run_time_configurable_transform_length=off  phase_factor_width=21  scaling_options=unscaled  rounding_modes=truncation  aclken=off  aresetn=off  output_ordering=natural_order  cyclic_prefix_insertion=off  throttle_scheme=nonrealtime  xk_index=off  ovflo=off  trim_axipin_name=on  memory_options_data=block_ram  memory_options_phase_factors=block_ram  number_of_stages_using_block_ram_for_data_and_phase_factors=3  memory_options_reorder=block_ram  memory_options_hybrid=off  complex_mult_type=use_mults_resources  butterfly_type=use_luts  simulation_type=hybrid_sim  simulation_model=sysgen:xfftv9_cmodel  data_path_portlist={ 's_axis_data_tdata', 'm_axis_data_tdata', 'm_axis_status_tdata', 'event_fft_overflow' }  channels=1  input_ordering=natural_order  input_width=16  ip_name=Fast Fourier Transform  ip_version=9.1  dsptool_ready=true  ipcore_usecache=true  ipcore_useipmodelcache=true  wrapper_available=true  port_translation_map={ 'aclken' => 'en', 'aresetn' => 'rst'}  data_format=fixed_point  block_type=xfft_v9_1
  Gateway In_i : xbsIndex_r4/Gateway In  gui_display_data_type=Fixed-point  arith_type="Signed  (2's comp)"  n_bits=12  bin_pt=11  preci_type=Single  exp_width=8  frac_width=24  rows=1  columns=1  quantization="Round  (unbiased: +/- Inf)"  overflow=Saturate  period=1/30720000  UseAsADC=off  ADCChannel='1'  interface=None  automatic_assignment=on  address_offset=hex2dec('00')  intf_name=''  intf_description=''  default_value=0  timing_constraint=None  locs_specified=off  LOCs={}  io_standard={}  inherit_from_input=off  hdl_port=on  dbl_ovrd=off  block_type=gatewayin
  Gateway In_q : xbsIndex_r4/Gateway In  gui_display_data_type=Fixed-point  arith_type="Signed  (2's comp)"  n_bits=12  bin_pt=11  preci_type=Single  exp_width=8  frac_width=24  rows=1  columns=1  quantization="Round  (unbiased: +/- Inf)"  overflow=Saturate  period=1/30720000  UseAsADC=off  ADCChannel='1'  interface=None  automatic_assignment=on  address_offset=hex2dec('00')  intf_name=''  intf_description=''  default_value=0  timing_constraint=None  locs_specified=off  LOCs={}  io_standard={}  inherit_from_input=off  hdl_port=on  dbl_ovrd=off  block_type=gatewayin
  Gateway N_loop : xbsIndex_r4/Gateway In  gui_display_data_type=Fixed-point  arith_type="Signed  (2's comp)"  n_bits=8  bin_pt=0  preci_type=Single  exp_width=8  frac_width=24  rows=1  columns=1  quantization="Round  (unbiased: +/- Inf)"  overflow=Saturate  period=1/30720000  UseAsADC=off  ADCChannel='1'  interface=None  automatic_assignment=on  address_offset=hex2dec('00')  intf_name=''  intf_description=''  default_value=0  timing_constraint=None  locs_specified=off  LOCs={}  io_standard={}  inherit_from_input=off  hdl_port=on  dbl_ovrd=off  block_type=gatewayin
  Gateway Out_data_sunc1 : xbsIndex_r4/Gateway Out  inherit_from_input=off  hdl_port=on  rows=1  columns=1  UseAsDAC=off  DACChannel='1'  interface=None  automatic_assignment=on  address_offset=hex2dec('00')  intf_name=''  intf_description=''  timing_constraint=None  locs_specified=off  LOCs={}  io_standard={}  block_type=gatewayout
  Gateway Out_data_sync_clk1 : xbsIndex_r4/Gateway Out  inherit_from_input=off  hdl_port=on  rows=1  columns=1  UseAsDAC=off  DACChannel='1'  interface=None  automatic_assignment=on  address_offset=hex2dec('00')  intf_name=''  intf_description=''  timing_constraint=None  locs_specified=off  LOCs={}  io_standard={}  block_type=gatewayout
  Gateway fur_mod : xbsIndex_r4/Gateway In  gui_display_data_type=Fixed-point  arith_type=Unsigned  n_bits=2  bin_pt=0  preci_type=Single  exp_width=8  frac_width=24  rows=1  columns=1  quantization="Round  (unbiased: +/- Inf)"  overflow=Saturate  period=1/30720000  UseAsADC=off  ADCChannel='1'  interface=None  automatic_assignment=on  address_offset=hex2dec('00')  intf_name=''  intf_description=''  default_value=0  timing_constraint=None  locs_specified=off  LOCs={}  io_standard={}  inherit_from_input=off  hdl_port=on  dbl_ovrd=off  block_type=gatewayin
  MATLAB Function 1 : MATLAB Function  TreatAsAtomicUnit=on
  MATLAB Function 2 : MATLAB Function  TreatAsAtomicUnit=on
  MATLAB Function 3 : MATLAB Function  TreatAsAtomicUnit=on
  "MCode " : xbsIndex_r4/MCode  mfname=quadrature_detector  explicit_period=off  period=1  inputsTable={'boundInpExpr'=>['','','','',''],'inputs'=>['i','q','s','c','e']}  outputsTable={'outputs'=>['i_out','q_out'],'suppressOut'=>['off','off']}  enable_stdout=off  enable_debug=off  suppress_output=on  defparams={}  hide_port_list={}  dbl_ovrd=off  block_type=mcode
  MCode2 : xbsIndex_r4/MCode  mfname=green_day  explicit_period=off  period=1  inputsTable={'boundInpExpr'=>['','',''],'inputs'=>['i','q','clok']}  outputsTable={'outputs'=>['i_out','q_out','plas','symma','flager','out_all','coun','regim'],'suppressOut'=>['off','off','off','off','off','off','off','off']}  enable_stdout=off  enable_debug=off  suppress_output=on  defparams={}  hide_port_list={}  dbl_ovrd=off  block_type=mcode
  "MCode2 " : xbsIndex_r4/MCode  mfname=fft_sum  explicit_period=off  period=1  inputsTable={'boundInpExpr'=>['','','',''],'inputs'=>['x','y','i','l']}  outputsTable={'outputs'=>['z','t'],'suppressOut'=>['off','off']}  enable_stdout=off  enable_debug=off  suppress_output=on  defparams={}  hide_port_list={}  dbl_ovrd=off  block_type=mcode
  MCode2 2 : xbsIndex_r4/MCode  mfname=fft_max_orig  explicit_period=off  period=1  inputsTable={'boundInpExpr'=>['',''],'inputs'=>['x','y']}  outputsTable={'outputs'=>['N','pinc','Bufe','Bufe_sr'],'suppressOut'=>['off','off','off','off']}  enable_stdout=off  enable_debug=off  suppress_output=on  defparams={}  hide_port_list={}  dbl_ovrd=off  block_type=mcode
  MCode4 : xbsIndex_r4/MCode  mfname=oqpsk_mult  explicit_period=off  period=1  inputsTable={'boundInpExpr'=>['','','','',''],'inputs'=>['i','q','i_o','q_o','regim']}  outputsTable={'outputs'=>['i_out','q_out'],'suppressOut'=>['off','off']}  enable_stdout=off  enable_debug=off  suppress_output=on  defparams={}  hide_port_list={}  dbl_ovrd=off  block_type=mcode
  MCode5 : xbsIndex_r4/MCode  mfname=symb_sync_500  explicit_period=off  period=1  inputsTable={'boundInpExpr'=>['',''],'inputs'=>['bit_in','bit_in2']}  outputsTable={'outputs'=>['data_sync','data_sync_2','data_sync_clk'],'suppressOut'=>['off','off','off']}  enable_stdout=off  enable_debug=off  suppress_output=on  defparams={}  hide_port_list={}  dbl_ovrd=off  block_type=mcode
  MCode6 1 : xbsIndex_r4/MCode  mfname=symb_sync_500_2  explicit_period=off  period=1  inputsTable={'boundInpExpr'=>[''],'inputs'=>['bit_in']}  outputsTable={'outputs'=>['data_sync','data_sync_clk'],'suppressOut'=>['off','off']}  enable_stdout=off  enable_debug=off  suppress_output=on  defparams={}  hide_port_list={}  dbl_ovrd=off  block_type=mcode
  MCode8 1 : xbsIndex_r4/MCode  mfname=costas4  explicit_period=off  period=1/30.72e6  inputsTable={'boundInpExpr'=>['',''],'inputs'=>['im','qm']}  outputsTable={'outputs'=>['im_out','qm_out'],'suppressOut'=>['off','off']}  enable_stdout=off  enable_debug=off  suppress_output=on  defparams={}  hide_port_list={}  dbl_ovrd=off  block_type=mcode
  MCode8 2 : xbsIndex_r4/MCode  mfname=quadrature_detector  explicit_period=off  period=1/30.72e6  inputsTable={'boundInpExpr'=>['','','','',''],'inputs'=>['i','q','s','c','e']}  outputsTable={'outputs'=>['i_out','q_out'],'suppressOut'=>['off','off']}  enable_stdout=off  enable_debug=off  suppress_output=on  defparams={}  hide_port_list={}  dbl_ovrd=off  block_type=mcode
  MCode8 3 : xbsIndex_r4/MCode  mfname=dds  explicit_period=off  period=1/30.72e6  inputsTable={'boundInpExpr'=>['','','',''],'inputs'=>['looper','furie','flag','fur_mod']}  outputsTable={'outputs'=>['z'],'suppressOut'=>['off']}  enable_stdout=off  enable_debug=off  suppress_output=on  defparams={}  hide_port_list={}  dbl_ovrd=off  block_type=mcode
  Manual Switch : ManualSwitch
  Manual Switch1 : ManualSwitch
  Mult1 : xbsIndex_r4/Mult  precision=User Defined  arith_type="Signed  (2's comp)"  n_bits=48  bin_pt=48  quantization=Truncate  overflow=Wrap  en=off  latency=1  use_behavioral_HDL=off  opt=Speed  use_embedded=on  optimum_pipeline=off  pipeline=on  dbl_ovrd=off  use_rpm=on  placement_style=Triangular  block_type=mult
  Mult2 : xbsIndex_r4/Mult  precision=Full  arith_type="Signed  (2's comp)"  n_bits=16  bin_pt=14  quantization=Truncate  overflow=Wrap  en=off  latency=0  use_behavioral_HDL=off  opt=Speed  use_embedded=on  optimum_pipeline=off  pipeline=on  dbl_ovrd=off  use_rpm=on  placement_style=Triangular  block_type=mult
  Mult3 : xbsIndex_r4/Mult  precision=Full  arith_type="Signed  (2's comp)"  n_bits=16  bin_pt=14  quantization=Truncate  overflow=Wrap  en=off  latency=0  use_behavioral_HDL=off  opt=Speed  use_embedded=on  optimum_pipeline=off  pipeline=on  dbl_ovrd=off  use_rpm=on  placement_style=Triangular  block_type=mult
  Mult4 : xbsIndex_r4/Mult  precision=User Defined  arith_type="Signed  (2's comp)"  n_bits=48  bin_pt=48  quantization=Truncate  overflow=Wrap  en=off  latency=1  use_behavioral_HDL=off  opt=Speed  use_embedded=on  optimum_pipeline=off  pipeline=on  dbl_ovrd=off  use_rpm=on  placement_style=Triangular  block_type=mult
  PM Modulator Passband 1 : commanapbnd3/PM Modulator Passband  Fc=1000500  Ph=0  Kc=pi/4
      settings: SourceProductName=Communications System Toolbox  SourceProductBaseCode=CM
  PM Modulator Passband 2 : commanapbnd3/PM Modulator Passband  Fc=1075000  Ph=0  Kc=pi/4
      settings: SourceProductName=Communications System Toolbox  SourceProductBaseCode=CM
  PM Modulator Passband1 1 : commanapbnd3/PM Modulator Passband  Fc=1000500  Ph=3*pi/2  Kc=pi/4
      settings: SourceProductName=Communications System Toolbox  SourceProductBaseCode=CM
  PM Modulator Passband1 2 : commanapbnd3/PM Modulator Passband  Fc=1075000  Ph=3*pi/2  Kc=pi/4
      settings: SourceProductName=Communications System Toolbox  SourceProductBaseCode=CM
  Pulse Generator 1 : DiscretePulseGenerator  Period=120  PulseWidth=60  PhaseDelay=60  SampleTime=1/30720000
  Pulse Generator 2 : DiscretePulseGenerator  Period=120  PulseWidth=60  SampleTime=1/30720000
  Pulse Generator 3 : DiscretePulseGenerator  Period=120  PulseWidth=60  SampleTime=1/30720000
  Real-Imag to Complex1 : RealImagToComplex
  "Reinterpret1 " : xbsIndex_r4/Reinterpret  force_arith_type=on  arith_type="Signed  (2's comp)"  force_bin_pt=on  bin_pt=20  block_type=reinterpret
  "Reinterpret2 " : xbsIndex_r4/Reinterpret  force_arith_type=on  arith_type="Signed  (2's comp)"  force_bin_pt=on  bin_pt=20  block_type=reinterpret
  Scope 1 : Scope
  Scope1 2 : Scope  NumInputPorts=3
  Scope1 3 : Scope  NumInputPorts=3
  Scope_cic1 : Scope
  Scope_cic2 : Scope
  Scope_dds{,2,5,7..13,17} (11 alike) : Scope
  Scope_dds{1,3..4,14} (4 alike) : Scope  NumInputPorts=2
  Scope_dds15 : Scope  NumInputPorts=3
  Scope_dds36 : Scope  NumInputPorts=3
  "Scope_fft " : Scope  NumInputPorts=2
  "Scope_fft_i " : Scope
  "Scope_fft_q " : Scope
  Scope_fir{1..4} (4 alike) : Scope
  "Slice1 " : xbsIndex_r4/Slice  nbits=21  boolean_output=off  mode=Upper Bit Location + Width  bit1=0  base1=MSB of Input  bit0=0  base0=LSB of Input  dbl_ovrd=off  block_type=slice
  "Slice3 " : xbsIndex_r4/Slice  nbits=21  boolean_output=off  mode=Upper Bit Location + Width  bit1=0  base1=MSB of Input  bit0=0  base0=LSB of Input  dbl_ovrd=off  block_type=slice
  Slice5 2 : xbsIndex_r4/Slice  nbits=1  boolean_output=off  mode=Upper Bit Location + Width  bit1=0  base1=MSB of Input  bit0=0  base0=LSB of Input  dbl_ovrd=off  block_type=slice
  Slice5 3 : xbsIndex_r4/Slice  nbits=1  boolean_output=off  mode=Upper Bit Location + Width  bit1=0  base1=MSB of Input  bit0=0  base0=LSB of Input  dbl_ovrd=off  block_type=slice
  Up Sample : xbsIndex_r4/Up Sample  sample_ratio=4  copy_samples=off  en=off  latency=1  dbl_ovrd=off  block_type=usamp
  bufferio : xbsIndex_r4/Gateway Out  inherit_from_input=off  hdl_port=on  rows=1  columns=1  UseAsDAC=off  DACChannel='1'  interface=None  automatic_assignment=on  address_offset=hex2dec('00')  intf_name=''  intf_description=''  timing_constraint=None  locs_specified=off  LOCs={}  io_standard={}  block_type=gatewayout
  bufferio_sr : xbsIndex_r4/Gateway Out  inherit_from_input=off  hdl_port=on  rows=1  columns=1  UseAsDAC=off  DACChannel='1'  interface=None  automatic_assignment=on  address_offset=hex2dec('00')  intf_name=''  intf_description=''  timing_constraint=None  locs_specified=off  LOCs={}  io_standard={}  block_type=gatewayout
  cic_out_1 : xbsIndex_r4/Gateway Out  inherit_from_input=off  hdl_port=off  rows=1  columns=1  UseAsDAC=off  DACChannel='1'  interface=None  automatic_assignment=on  address_offset=hex2dec('00')  intf_name=''  intf_description=''  timing_constraint=None  locs_specified=off  LOCs={}  io_standard={}  block_type=gatewayout
  cic_out_2 : xbsIndex_r4/Gateway Out  inherit_from_input=off  hdl_port=off  rows=1  columns=1  UseAsDAC=off  DACChannel='1'  interface=None  automatic_assignment=on  address_offset=hex2dec('00')  intf_name=''  intf_description=''  timing_constraint=None  locs_specified=off  LOCs={}  io_standard={}  block_type=gatewayout
  cos_dds : xbsIndex_r4/Gateway Out  inherit_from_input=off  hdl_port=off  rows=1  columns=1  UseAsDAC=off  DACChannel='1'  interface=None  automatic_assignment=on  address_offset=hex2dec('00')  intf_name=''  intf_description=''  timing_constraint=None  locs_specified=off  LOCs={}  io_standard={}  block_type=gatewayout
  data_sync1 : xbsIndex_r4/Gateway Out  inherit_from_input=off  hdl_port=on  rows=1  columns=1  UseAsDAC=off  DACChannel='1'  interface=None  automatic_assignment=on  address_offset=hex2dec('00')  intf_name=''  intf_description=''  timing_constraint=None  locs_specified=off  LOCs={}  io_standard={}  block_type=gatewayout
  data_sync_1 : xbsIndex_r4/Gateway Out  inherit_from_input=off  hdl_port=on  rows=1  columns=1  UseAsDAC=off  DACChannel='1'  interface=None  automatic_assignment=on  address_offset=hex2dec('00')  intf_name=''  intf_description=''  timing_constraint=None  locs_specified=off  LOCs={}  io_standard={}  block_type=gatewayout
  data_sync_clk1 : xbsIndex_r4/Gateway Out  inherit_from_input=off  hdl_port=on  rows=1  columns=1  UseAsDAC=off  DACChannel='1'  interface=None  automatic_assignment=on  address_offset=hex2dec('00')  intf_name=''  intf_description=''  timing_constraint=None  locs_specified=off  LOCs={}  io_standard={}  block_type=gatewayout
  fft_spector : xbsIndex_r4/Gateway Out  inherit_from_input=off  hdl_port=on  rows=1  columns=1  UseAsDAC=off  DACChannel='1'  interface=None  automatic_assignment=on  address_offset=hex2dec('00')  intf_name=''  intf_description=''  timing_constraint=None  locs_specified=off  LOCs={}  io_standard={}  block_type=gatewayout
  fft_tlast : xbsIndex_r4/Gateway Out  inherit_from_input=off  hdl_port=on  rows=1  columns=1  UseAsDAC=off  DACChannel='1'  interface=None  automatic_assignment=on  address_offset=hex2dec('00')  intf_name=''  intf_description=''  timing_constraint=None  locs_specified=off  LOCs={}  io_standard={}  block_type=gatewayout
  fir_out_{1..4} (4 alike) : xbsIndex_r4/Gateway Out  inherit_from_input=off  hdl_port=off  rows=1  columns=1  UseAsDAC=off  DACChannel='1'  interface=None  automatic_assignment=on  address_offset=hex2dec('00')  intf_name=''  intf_description=''  timing_constraint=None  locs_specified=off  LOCs={}  io_standard={}  block_type=gatewayout
  flag1 : xbsIndex_r4/Gateway Out  inherit_from_input=off  hdl_port=on  rows=1  columns=1  UseAsDAC=off  DACChannel='1'  interface=None  automatic_assignment=on  address_offset=hex2dec('00')  intf_name=''  intf_description=''  timing_constraint=None  locs_specified=off  LOCs={}  io_standard={}  block_type=gatewayout
  i_bit_slice : xbsIndex_r4/Gateway Out  inherit_from_input=off  hdl_port=on  rows=1  columns=1  UseAsDAC=off  DACChannel='1'  interface=None  automatic_assignment=on  address_offset=hex2dec('00')  intf_name=''  intf_description=''  timing_constraint=None  locs_specified=off  LOCs={}  io_standard={}  block_type=gatewayout
  i_bit_slice_symb1 : xbsIndex_r4/Gateway Out  inherit_from_input=off  hdl_port=on  rows=1  columns=1  UseAsDAC=off  DACChannel='1'  interface=None  automatic_assignment=on  address_offset=hex2dec('00')  intf_name=''  intf_description=''  timing_constraint=None  locs_specified=off  LOCs={}  io_standard={}  block_type=gatewayout
  "i_in_fft " : xbsIndex_r4/Gateway Out  inherit_from_input=off  hdl_port=off  rows=1  columns=1  UseAsDAC=off  DACChannel='1'  interface=None  automatic_assignment=on  address_offset=hex2dec('00')  intf_name=''  intf_description=''  timing_constraint=None  locs_specified=off  LOCs={}  io_standard={}  block_type=gatewayout
  i_oqpsk_mult : xbsIndex_r4/Gateway Out  inherit_from_input=off  hdl_port=on  rows=1  columns=1  UseAsDAC=off  DACChannel='1'  interface=None  automatic_assignment=on  address_offset=hex2dec('00')  intf_name=''  intf_description=''  timing_constraint=None  locs_specified=off  LOCs={}  io_standard={}  block_type=gatewayout
  in_i : xbsIndex_r4/Gateway Out  inherit_from_input=off  hdl_port=on  rows=1  columns=1  UseAsDAC=off  DACChannel='1'  interface=None  automatic_assignment=on  address_offset=hex2dec('00')  intf_name=''  intf_description=''  timing_constraint=None  locs_specified=off  LOCs={}  io_standard={}  block_type=gatewayout
  in_i_fir : xbsIndex_r4/Gateway Out  inherit_from_input=off  hdl_port=on  rows=1  columns=1  UseAsDAC=off  DACChannel='1'  interface=None  automatic_assignment=on  address_offset=hex2dec('00')  intf_name=''  intf_description=''  timing_constraint=None  locs_specified=off  LOCs={}  io_standard={}  block_type=gatewayout
  in_q : xbsIndex_r4/Gateway Out  inherit_from_input=off  hdl_port=on  rows=1  columns=1  UseAsDAC=off  DACChannel='1'  interface=None  automatic_assignment=on  address_offset=hex2dec('00')  intf_name=''  intf_description=''  timing_constraint=None  locs_specified=off  LOCs={}  io_standard={}  block_type=gatewayout
  in_q_fir : xbsIndex_r4/Gateway Out  inherit_from_input=off  hdl_port=on  rows=1  columns=1  UseAsDAC=off  DACChannel='1'  interface=None  automatic_assignment=on  address_offset=hex2dec('00')  intf_name=''  intf_description=''  timing_constraint=None  locs_specified=off  LOCs={}  io_standard={}  block_type=gatewayout
  n_fft : xbsIndex_r4/Gateway Out  inherit_from_input=off  hdl_port=on  rows=1  columns=1  UseAsDAC=off  DACChannel='1'  interface=None  automatic_assignment=on  address_offset=hex2dec('00')  intf_name=''  intf_description=''  timing_constraint=None  locs_specified=off  LOCs={}  io_standard={}  block_type=gatewayout
  out_posl1 : xbsIndex_r4/Gateway Out  inherit_from_input=off  hdl_port=on  rows=1  columns=1  UseAsDAC=off  DACChannel='1'  interface=None  automatic_assignment=on  address_offset=hex2dec('00')  intf_name=''  intf_description=''  timing_constraint=None  locs_specified=off  LOCs={}  io_standard={}  block_type=gatewayout
  "pinc_fft " : xbsIndex_r4/Gateway Out  inherit_from_input=off  hdl_port=off  rows=1  columns=1  UseAsDAC=off  DACChannel='1'  interface=None  automatic_assignment=on  address_offset=hex2dec('00')  intf_name=''  intf_description=''  timing_constraint=None  locs_specified=off  LOCs={}  io_standard={}  block_type=gatewayout
  polozhenie_green : xbsIndex_r4/Gateway Out  inherit_from_input=off  hdl_port=on  rows=1  columns=1  UseAsDAC=off  DACChannel='1'  interface=None  automatic_assignment=on  address_offset=hex2dec('00')  intf_name=''  intf_description=''  timing_constraint=None  locs_specified=off  LOCs={}  io_standard={}  block_type=gatewayout
  q_bit_slice : xbsIndex_r4/Gateway Out  inherit_from_input=off  hdl_port=on  rows=1  columns=1  UseAsDAC=off  DACChannel='1'  interface=None  automatic_assignment=on  address_offset=hex2dec('00')  intf_name=''  intf_description=''  timing_constraint=None  locs_specified=off  LOCs={}  io_standard={}  block_type=gatewayout
  q_bit_slice_symb1 : xbsIndex_r4/Gateway Out  inherit_from_input=off  hdl_port=on  rows=1  columns=1  UseAsDAC=off  DACChannel='1'  interface=None  automatic_assignment=on  address_offset=hex2dec('00')  intf_name=''  intf_description=''  timing_constraint=None  locs_specified=off  LOCs={}  io_standard={}  block_type=gatewayout
  "q_in_fft " : xbsIndex_r4/Gateway Out  inherit_from_input=off  hdl_port=off  rows=1  columns=1  UseAsDAC=off  DACChannel='1'  interface=None  automatic_assignment=on  address_offset=hex2dec('00')  intf_name=''  intf_description=''  timing_constraint=None  locs_specified=off  LOCs={}  io_standard={}  block_type=gatewayout
  q_oqpsk_mult : xbsIndex_r4/Gateway Out  inherit_from_input=off  hdl_port=on  rows=1  columns=1  UseAsDAC=off  DACChannel='1'  interface=None  automatic_assignment=on  address_offset=hex2dec('00')  intf_name=''  intf_description=''  timing_constraint=None  locs_specified=off  LOCs={}  io_standard={}  block_type=gatewayout
  regim_oqpsk : xbsIndex_r4/Gateway Out  inherit_from_input=off  hdl_port=on  rows=1  columns=1  UseAsDAC=off  DACChannel='1'  interface=None  automatic_assignment=on  address_offset=hex2dec('00')  intf_name=''  intf_description=''  timing_constraint=None  locs_specified=off  LOCs={}  io_standard={}  block_type=gatewayout
  sin_dds {,1..3,7..9,14} (8 alike) : xbsIndex_r4/Gateway Out  inherit_from_input=off  hdl_port=off  rows=1  columns=1  UseAsDAC=off  DACChannel='1'  interface=None  automatic_assignment=on  address_offset=hex2dec('00')  intf_name=''  intf_description=''  timing_constraint=None  locs_specified=off  LOCs={}  io_standard={}  block_type=gatewayout
  wires:
  "Constant1 "/1 -> "Fast Fourier Transform 9.1 "/2, "Fast Fourier Transform 9.1 "/5, "Fast Fourier Transform 9.1 "/6, "Fast Fourier Transform 9.1 "/7
  "Down Sample7 "/1 -> "Slice1 "/1
  "Reinterpret2 "/1 -> "Fast Fourier Transform 9.1 "/3
  "CIC Compiler 4.0 2 "/3 -> "Down Sample2 "/1, cic_out_2/1
  "Fast Fourier Transform 9.1 "/6 -> "MCode2 "/4
  "CIC Compiler 4.0 2 "/2 -> "FIR Compiler 7.2 3 "/1
  "Down Sample2 "/1 -> "FIR Compiler 7.2 3 "/2
  "MCode "/2 -> "CIC Compiler 4.0 1 "/2, "q_in_fft "/1
  "Constant2 "/1 -> "Fast Fourier Transform 9.1 "/1
  Constant11 5/1 -> DDS Compiler 6.0 2 1/1
  "MCode2 "/1 -> MCode2 2/1, fft_spector/1
  "CIC Compiler 4.0 1 "/3 -> "Down Sample1 "/1, cic_out_1/1
  "Down Sample1 "/1 -> "FIR Compiler 7.2 1 "/2
  "Reinterpret1 "/1 -> "Fast Fourier Transform 9.1 "/4
  "Convert1 "/1 -> "Reinterpret2 "/1
  "Fast Fourier Transform 9.1 "/3 -> "MCode2 "/1, fir_out_3/1
  "q_in_fft "/1 -> "Scope_fft_q "/1
  "Convert "/1 -> "Reinterpret1 "/1
  "CIC Compiler 4.0 1 "/2 -> "FIR Compiler 7.2 1 "/1
  "i_in_fft "/1 -> "Scope_fft_i "/1
  "Down Sample6 "/1 -> "Slice3 "/1
  fir_out_2/1 -> Scope_fir2/1
  cos_dds/1 -> Scope_dds5/1
  "MCode "/1 -> "CIC Compiler 4.0 2 "/2, "i_in_fft "/1
  fft_tlast/1 -> "Scope_fft "/2
  cic_out_1/1 -> Scope_cic1/1
  "Slice3 "/1 -> "Convert1 "/1
  "sin_dds "/1 -> Scope_dds/1
  "Fast Fourier Transform 9.1 "/5 -> "MCode2 "/3
  fir_out_4/1 -> Scope_fir4/1
  fir_out_3/1 -> Scope_fir3/1
  "Fast Fourier Transform 9.1 "/4 -> "MCode2 "/2, fir_out_4/1
  "FIR Compiler 7.2 1 "/3 -> "Down Sample6 "/1, fir_out_1/1
  "FIR Compiler 7.2 3 "/3 -> fir_out_2/1, "Down Sample7 "/1
  "Slice1 "/1 -> "Convert "/1
  fir_out_1/1 -> Scope_fir1/1
  fft_spector/1 -> "Scope_fft "/1
  DDS Compiler 6.0 2 1/3 -> "sin_dds "/1, "MCode "/3
  cic_out_2/1 -> Scope_cic2/1
  DDS Compiler 6.0 2 1/4 -> cos_dds/1, "MCode "/4
  DDS Compiler 6.0 2 1/2 -> "MCode "/5, "CIC Compiler 4.0 2 "/1, "CIC Compiler 4.0 1 "/1
  Constant10 1/1 -> DDS Compiler 6.0 2 1/4
  Constant11 7/1 -> DDS Compiler 6.0 2 1/2
  Constant9 1/1 -> DDS Compiler 6.0 2 1/3
  in_q/1 -> Scope_dds10/1
  MCode8 3/1 -> sin_dds 3/1, DDS Compiler 6.0 2 2/2
  Mult3/1 -> AddSub2/2
  in_i/1 -> Scope_dds9/1
  PM Modulator Passband1 2/1 -> Scope_dds1/2, Manual Switch1/1
  Delay1 2/1 -> AddSub3 2/2
  FIR Compiler 7.2 2 4/3 -> Slice5 2/1, in_q_fir/1
  MCode5/1 -> MCode2/1, data_sync1/1
  Gateway In_q/1 -> MCode8 2/2, "MCode "/2
  AddSub2 2/1 -> MCode8 3/1, sin_dds 2/1
  in_q_fir/1 -> Scope_dds13/1, Real-Imag to Complex1/2
  MCode2/6 -> sin_dds 9/1, out_posl1/1, MCode6 1/1
  MCode8 1/2 -> sin_dds 1/1, Mult2/2
  Down Sample4 4/1 -> FIR Compiler 7.2 2 4/2
  PM Modulator Passband 2/1 -> Scope_dds1/1, Manual Switch/1
  MATLAB Function 1/1(y) -> PM Modulator Passband1 2/1, Scope_dds4/2
  MCode8 2/2 -> MCode8 1/2, Mult3/1, CIC Compiler 4.0 4 4/2, in_q/1
  Mult2/1 -> AddSub2/1
  DDS Compiler 6.0 2 2/2 -> Delay1 2/2, CIC Compiler 4.0 4 1/1, CIC Compiler 4.0 4 4/1, MCode8 2/5
  sin_dds 1/1 -> Display6/1
  Constant10 2/1 -> DDS Compiler 6.0 2 2/4
  Constant9 2/1 -> DDS Compiler 6.0 2 2/3
  i_bit_slice/1 -> Scope_dds36/1
  Down Sample4 1/1 -> FIR Compiler 7.2 2 1/2
  DDS Compiler 6.0 2 2/4 -> MCode8 2/4
  DDS Compiler 6.0 2 2/3 -> MCode8 2/3
  data_sync_1/1 -> Scope_dds15/2
  in_i_fir/1 -> Scope_dds12/1, Real-Imag to Complex1/1
  CIC Compiler 4.0 4 1/3 -> Down Sample4 1/1
  CIC Compiler 4.0 4 1/2 -> FIR Compiler 7.2 2 1/1
  MATLAB Function 3/1(y) -> PM Modulator Passband 1/1, PM Modulator Passband1 1/1, Scope_dds7/1
  MCode8 2/1 -> Mult2/1, MCode8 1/1, CIC Compiler 4.0 4 1/2, in_i/1
  MCode8 1/1 -> Mult3/2, sin_dds 14/1
  Pulse Generator 2/1 -> MATLAB Function 3/1(u)
  FIR Compiler 7.2 2 1/3 -> Slice5 3/1, in_i_fir/1
  Manual Switch1/1 -> Gateway In_q/1
  CIC Compiler 4.0 4 4/2 -> FIR Compiler 7.2 2 4/1
  Real-Imag to Complex1/1 -> Constellation Diagram1/1
  flag1/1 -> Display3/1, Scope1 3/3, Scope_dds17/1
  Gateway Out_data_sync_clk1/1 -> Scope1 2/1
  PM Modulator Passband 1/1 -> Scope_dds8/1, Manual Switch/2
  data_sync1/1 -> Scope_dds15/1
  Pulse Generator 3/1 -> MATLAB Function 2/1(u)
  q_bit_slice/1 -> Scope_dds36/2
  polozhenie_green/1 -> Display4/1
  MCode2/7 -> sin_dds 8/1
  MCode2/8 -> regim_oqpsk/1, Delay3/1
  AddSub3 2/1 -> AddSub2 2/2, Delay1 2/1
  MCode2/5 -> MCode8 3/3, flag1/1
  regim_oqpsk/1 -> Display7/1
  MCode4/1 -> i_oqpsk_mult/1, MCode5/1
  Delay1/1 -> MCode4/3
  Manual Switch/1 -> Gateway In_i/1
  MCode2/4 -> sin_dds 7/1
  MCode6 1/2 -> Gateway Out_data_sync_clk1/1
  Pulse Generator 1/1 -> MATLAB Function 1/1(u)
  CIC Compiler 4.0 4 4/3 -> Down Sample4 4/1
  sin_dds 14/1 -> Display5/1
  MCode2/2 -> q_bit_slice_symb1/1
  q_bit_slice_symb1/1 -> Scope_dds14/2
  MCode5/3 -> MCode2/3, data_sync_clk1/1
  Gateway In_i/1 -> MCode8 2/1, "MCode "/1
  sin_dds 9/1 -> Scope1 3/1
  sin_dds 8/1 -> Scope1 3/2
  MATLAB Function 2/1(y) -> PM Modulator Passband 2/1, Scope_dds4/1
  out_posl1/1 -> Scope_dds11/1, Scope1 2/3
  Gateway Out_data_sunc1/1 -> Scope 1/1, Scope1 2/2
  Delay2/1 -> MCode4/4
  i_bit_slice_symb1/1 -> Scope_dds14/1
  Constant11 2/1 -> DDS Compiler 6.0 2 2/1
  MCode2/1 -> i_bit_slice_symb1/1
  MCode2/3 -> polozhenie_green/1
  Slice5 3/1 -> i_bit_slice/1, MCode4/1, Delay1/1
  MCode4/2 -> q_oqpsk_mult/1, MCode5/2
  Delay3/1 -> MCode4/5
  MCode6 1/1 -> Gateway Out_data_sunc1/1
  MCode5/2 -> MCode2/2, data_sync_1/1
  Slice5 2/1 -> q_bit_slice/1, MCode4/2, Delay2/1
  sin_dds 7/1 -> Display8/1
  PM Modulator Passband1 1/1 -> Manual Switch1/2
  data_sync_clk1/1 -> Scope_dds15/3
  "MCode2 "/2 -> MCode2 2/2, fft_tlast/1
  n_fft/1 -> "Display5 "/1
  "pinc_fft "/1 -> "Display4 "/1
  MCode2 2/2 -> Up Sample/1, "pinc_fft "/1
  MCode2 2/1 -> n_fft/1
  bufferio/1 -> Display5 1/1
  MCode2 2/3 -> bufferio/1
  MCode2 2/4 -> bufferio_sr/1
  bufferio_sr/1 -> Display5 2/1
  CMult4 5/1 -> Mult1/1
  Gateway N_loop/1 -> Mult4/2, Mult1/2
  Constant2/1 -> Gateway N_loop/1
  CMult3 5/1 -> Mult4/1
  Mult4/1 -> AddSub3 2/1
  Mult1/1 -> AddSub2 2/1
  AddSub2/1 -> CMult3 5/1, CMult4 5/1
  Up Sample/1 -> MCode8 3/2
  Gateway fur_mod/1 -> MCode8 3/4
  Constant1/1 -> Gateway fur_mod/1
  sin_dds 2/1 -> Scope_dds2/1
  sin_dds 3/1 -> Display1/1
  i_oqpsk_mult/1 -> Scope_dds3/1
  q_oqpsk_mult/1 -> Scope_dds3/2
